simulink model "homework_b_c"  (R2025a)
settings: Solver=VariableStepAuto  StartTime=0.0  StopTime=30  RelTol=1e-3
settings Model: Creator=Admin  LastModifiedBy=Admin

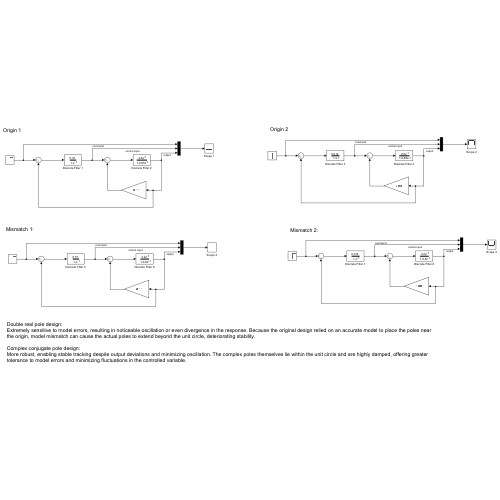
[thumbnail: Simulink's stored preview of the top-level diagram]
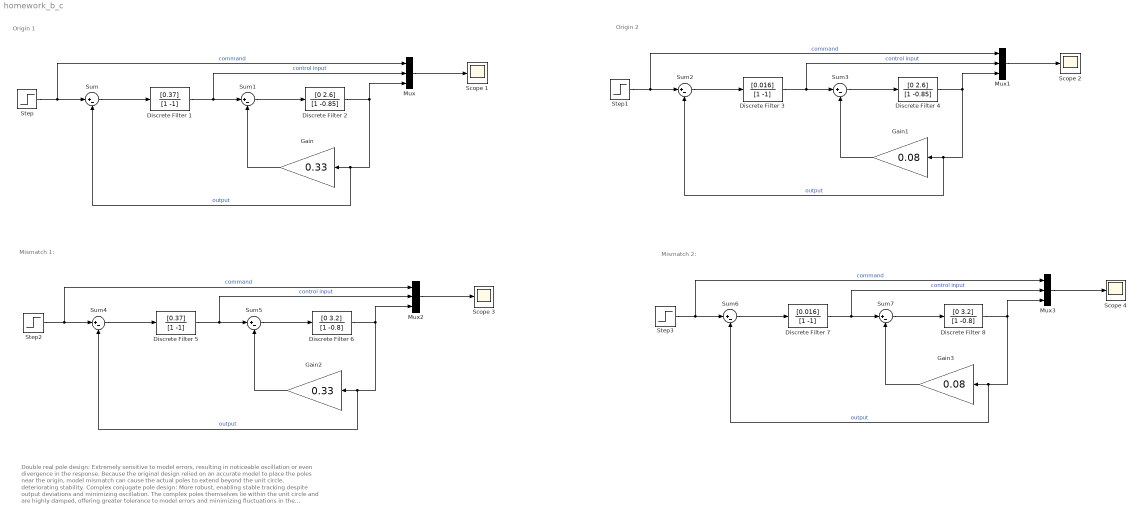
== system homework_b_c ==
  note: Double real pole design:
      | Extremely sensitive to model errors, resulting in noticeable oscillation or even divergence in the response. Because the original design relied on an accurate model to place the poles near the origin, model mismatch can cause the actual poles to extend beyond the unit circle, deteriorating stability.
      |
      | Complex conjugate pole design:
      | More robust, enabling stable tracking despite output deviations and minimizing oscillation. The complex poles themselves lie within the unit circle and are highly damped, offering greater tolerance to model errors and minimizing fluctuations in the controlled variable.
  note: Origin 2
  note: Origin 1
  note: Mismatch 1:
  note: Mismatch 2:
  Discrete Filter 1 : DiscreteFilter  Numerator=[0.37]  Denominator=[1 -1]
  Discrete Filter 2 : DiscreteFilter  Numerator=[0 2.6]  Denominator=[1 -0.85]
  Discrete Filter 3 : DiscreteFilter  Numerator=[0.016]  Denominator=[1 -1]
  Discrete Filter 4 : DiscreteFilter  Numerator=[0 2.6]  Denominator=[1 -0.85]
  Discrete Filter 5 : DiscreteFilter  Numerator=[0.37]  Denominator=[1 -1]
  Discrete Filter 6 : DiscreteFilter  Numerator=[0 3.2]  Denominator=[1 -0.8]
  Discrete Filter 7 : DiscreteFilter  Numerator=[0.016]  Denominator=[1 -1]
  Discrete Filter 8 : DiscreteFilter  Numerator=[0 3.2]  Denominator=[1 -0.8]
  Gain : Gain  Gain=0.33
  Gain1 : Gain  Gain=0.08
  Gain2 : Gain  Gain=0.33
  Gain3 : Gain  Gain=0.08
  Mux{,1..3} (4 alike) : Mux  Inputs=3
  Scope {1..4} (4 alike) : Scope
      Scope 1 settings: ActiveDisplayYMinimum=-1.8590585292098878  ActiveDisplayYMaximum=1.8735614695179537
      Scope 2 settings: ActiveDisplayYMinimum=-0.34275370809302208  ActiveDisplayYMaximum=1.1098464207477092
      Scope 3 settings: ActiveDisplayYMinimum=-1.8590585292098878  ActiveDisplayYMaximum=1.8735614695179537  DataLoggingVariableName=ScopeData2
      Scope 4 settings: ActiveDisplayYMinimum=-0.34275370809302208  ActiveDisplayYMaximum=1.1098464207477092  DataLoggingVariableName=ScopeData3
  Step{,1..3} (4 alike) : Step  SampleTime=0
  Sum{,1..7} (8 alike) : Sum  Inputs=|+-
  wires:
  Sum/1 -> Discrete Filter 1/1
  Step/1 -> Mux/1, Sum/1  "command"
  Discrete Filter 1/1 -> Mux/2, Sum1/1  "control input"
  Sum1/1 -> Discrete Filter 2/1
  Discrete Filter 2/1 -> Sum/2, Gain/1, Mux/3  "output"
  Gain/1 -> Sum1/2
  Mux/1 -> Scope 1/1
  Discrete Filter 4/1 -> Sum2/2, Gain1/1, Mux1/3  "output"
  Sum3/1 -> Discrete Filter 4/1
  Step1/1 -> Mux1/1, Sum2/1  "command"
  Gain1/1 -> Sum3/2
  Discrete Filter 3/1 -> Mux1/2, Sum3/1  "control input"
  Mux1/1 -> Scope 2/1
  Sum2/1 -> Discrete Filter 3/1
  Step2/1 -> Mux2/1, Sum4/1  "command"
  Discrete Filter 5/1 -> Mux2/2, Sum5/1  "control input"
  Discrete Filter 6/1 -> Sum4/2, Gain2/1, Mux2/3  "output"
  Sum5/1 -> Discrete Filter 6/1
  Mux2/1 -> Scope 3/1
  Gain2/1 -> Sum5/2
  Sum4/1 -> Discrete Filter 5/1
  Sum6/1 -> Discrete Filter 7/1
  Step3/1 -> Mux3/1, Sum6/1  "command"
  Discrete Filter 7/1 -> Mux3/2, Sum7/1  "control input"
  Gain3/1 -> Sum7/2
  Discrete Filter 8/1 -> Sum6/2, Gain3/1, Mux3/3  "output"
  Mux3/1 -> Scope 4/1
  Sum7/1 -> Discrete Filter 8/1
